simulink model "VDP_OSCILLATOR"  (Simulink 8.3)
settings: Solver=ode5  StartTime=0.0  StopTime=T  FixedStep=1/Fs  RelTol=1e-3
values from neighbouring files (symbols this model uses):
  alpha = alpha_i(ii)    [Self_study_lesson_stochastic_oscillator.m]
  beta = 60    [Self_study_lesson_stochastic_oscillator.m]
  Fs = 1000    [Self_study_lesson_stochastic_oscillator.m]
  kappa = 3.4    [Self_study_lesson_stochastic_oscillator.m]
  wn = 2*pi*120    (= 753.982236862)    [Self_study_lesson_stochastic_oscillator.m]
libraries: simulink x1
settings Model: Creator=bschuerm  LastModifiedBy=noirayn  ExtModeAutoUpdateStatusClock=off
settings OptimizationCC: ExpressionDepthLimit=2147483647
settings DebuggingCC: SaveWithParameterizedLinksMsg=none  FcnCallInpInsideContextMsg=UseLocalSettings

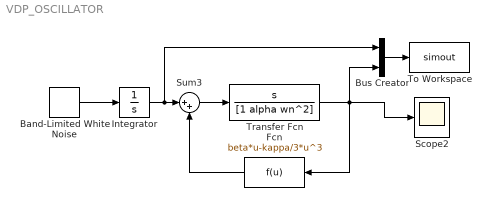
== system VDP_OSCILLATOR ==
  Band-Limited White Noise : simulink/Sources/Band-Limited White Noise  Cov=Gamma  Ts=1/Fs  seed=random_seed
  Bus Creator : BusCreator  Inputs=2
  Fcn : Fcn  Expr=beta*u-kappa/3*u^3
  Integrator : Integrator
  Scope2 : Scope
      settings: YMin=-10  YMax=10
  Sum3 : Sum  Inputs=|++
  To Workspace : ToWorkspace  VariableName=simout  SaveFormat=Structure With Time  SampleTime=-1
  Transfer Fcn : TransferFcn  Numerator=[1 0]  Denominator=[1 alpha wn^2]
  wires:
  Sum3/1 -> Transfer Fcn/1
  Transfer Fcn/1 -> Scope2/1, Bus Creator/2, Fcn/1
  Fcn/1 -> Sum3/2
  Band-Limited White Noise/1 -> Integrator/1
  Integrator/1 -> Bus Creator/1, Sum3/1
  Bus Creator/1 -> To Workspace/1
